simulink model "OtterFullForLqr_PositionControll_backup_LQR"  (R2020b)
settings: Solver=VariableStepAuto  StartTime=0.0  StopTime=30  RelTol=1e-3
values from neighbouring files (symbols this model uses):
  N = inv(Dcgain)    [LinMod60rpmForLqr.m]
  u0 = [60 60]'    [LinMod60rpmForLqr.m]
  x0 = OpTrim60.states.x    [LinMod60rpmForLqr.m]
undefined symbols (not defined in the file or in its folder): F
libraries: simulink x1, mssSimulink x1
settings Model: Creator=rapha  LastModifiedBy=rapha
settings DataIOCC: ExternalInput=getinputstruct(op_trim1)  InitialState=getstatestruct(op_trim1)

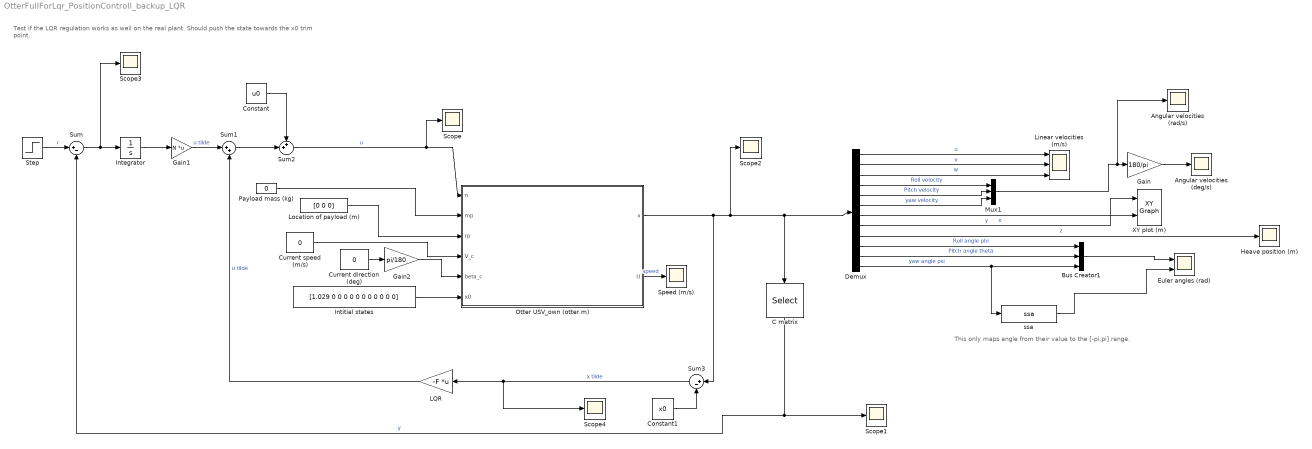
== system OtterFullForLqr_PositionControll_backup_LQR ==
  note: Test if the LQR regulation works as well on the real plant. Should push the state towards the x0 trim point.
  note: This only maps angle from their value to the [-pi,pi] range.
  Angular velocities (deg/s) : Scope
  Angular velocities (rad/s) : Scope
  Bus Creator1 : BusCreator  Inputs=3
  C matrix : Selector  InputPortWidth=12  IndexOptions=Index vector (dialog)  Indices=[1 6]  OutputSizes=1
  Constant : Constant  Value=u0
  Constant1 : Constant  Value=x0
  Current direction (deg) : Constant  Value=0
  Current speed (m/s) : Constant  Value=0
  Demux : Demux  Outputs=12
  Euler angles (rad) : Scope  NumInputPorts=2
  Gain : Gain  Gain=180/pi
  Gain1 : Gain  Gain=N  Multiplication=Matrix(K*u)
  Gain2 : Gain  Gain=pi/180
  Heave position (m) : Scope
  Integrator : Integrator
  Intitial states : Constant  Value=[1.029 0 0 0 0 0 0 0 0 0 0 0]
  LQR : Gain  Gain=-F  Multiplication=Matrix(K*u)
  Linear velocities (m/s) : Scope  NumInputPorts=3
  Location of payload (m) : Constant  Value=[0 0 0]
  Mux1 : Mux  Inputs=3
  "Otter USV_own (otter.m) " : Subsystem  AncestorBlock=mssSimulink/Marine craft models/Otter USV (otter.m)
      mask Display: image('otter.jpg'); % Use "Edit Image" on toolstrip to change.
  Payload mass (kg) : Constant  Value=0
  Scope{,1..4} (5 alike) : Scope
  Speed (m/s) : Scope
  Step : Step  Time=4  Before=[1.029 0]  After=[2 0.15]  SampleTime=0
  Sum : Sum  Inputs=|+-
  Sum1 : Sum  Inputs=|++
  Sum2 : Sum  Inputs=++|
  Sum3 : Sum  Inputs=|+-
  XY plot (m) : simulink/Sinks/XY Graph  xmin=-70  xmax=70  ymin=-70  ymax=70  st=0.01
  "ssa   " : mssSimulink/Utilities/Math Operations/ssa  SystemSampleTime=-1  VariantActivationTime=update diagram  Latency=0  AutoFrameSizeCalculation=off
  wires:
  Intitial states/1 -> "Otter USV_own (otter.m) "/6(x0)
  Payload mass (kg)/1 -> "Otter USV_own (otter.m) "/2(mp)
  Gain2/1 -> "Otter USV_own (otter.m) "/5(beta_c)
  Current direction (deg)/1 -> Gain2/1
  "Otter USV_own (otter.m) "/2(U) -> Speed (m/s)/1  "speed"
  Current speed (m/s)/1 -> "Otter USV_own (otter.m) "/4(V_c)
  Location of payload (m)/1 -> "Otter USV_own (otter.m) "/3(rp)
  Demux/1 -> Linear velocities (m/s)/1  "u"
  Demux/8 -> XY plot (m)/1  "y"
  Demux/7 -> XY plot (m)/2  "x"
  Demux/2 -> Linear velocities (m/s)/2  "v"
  Demux/3 -> Linear velocities (m/s)/3  "w"
  Gain/1 -> Angular velocities (deg/s)/1
  Mux1/1 -> Angular velocities (rad/s)/1, Gain/1
  Demux/4 -> Mux1/1  "Roll velocity"
  Demux/5 -> Mux1/2  "Pitch velocity"
  Demux/6 -> Mux1/3  "yaw velocity"
  Demux/9 -> Heave position (m)/1  "z"
  Demux/11 -> Bus Creator1/2  "Pitch angle theta"
  Bus Creator1/1 -> Euler angles (rad)/1
  Demux/10 -> Bus Creator1/1  "Roll angle phi"
  Demux/12 -> "ssa   "/1, Bus Creator1/3  "yaw angle psi"
  "ssa   "/1 -> Euler angles (rad)/2
  "Otter USV_own (otter.m) "/1(x) -> Sum3/1, C matrix/1, Demux/1, Scope2/1
  C matrix/1 -> Scope1/1, Sum/2  "y"
  Step/1 -> Sum/1  "r"
  Sum/1 -> Integrator/1, Scope3/1
  LQR/1 -> Sum1/2  "u tilde"
  Gain1/1 -> Sum1/1  "u tilde"
  Sum1/1 -> Sum2/2
  Sum2/1 -> Scope/1, "Otter USV_own (otter.m) "/1(n)  "u"
  Sum3/1 -> Scope4/1, LQR/1  "x tilde"
  Constant1/1 -> Sum3/2
  Constant/1 -> Sum2/1
  Integrator/1 -> Gain1/1

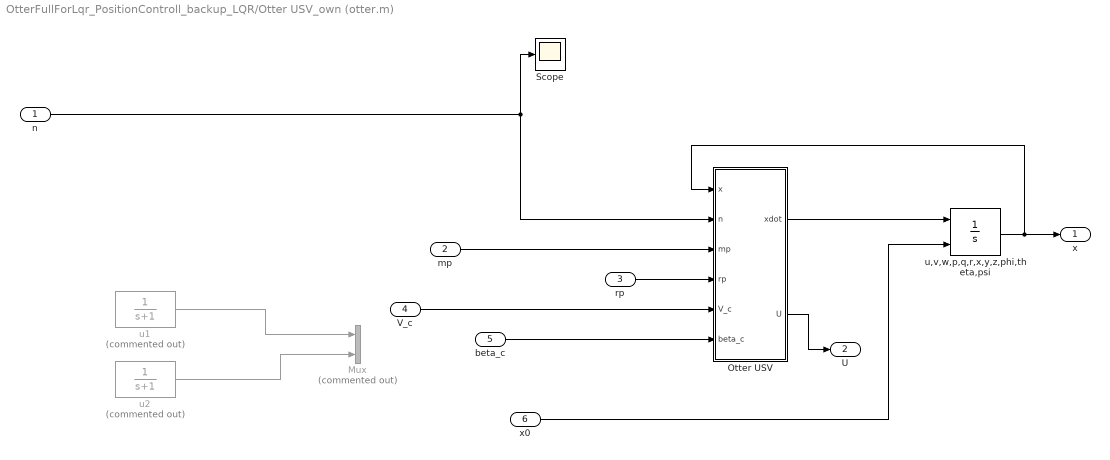
== system OtterFullForLqr_PositionControll_backup_LQR/Otter USV_own (otter.m)  ==
  n : Inport
  mp : Inport  Port=2
  rp : Inport  Port=3
  V_c : Inport  Port=4
  beta_c : Inport  Port=5
  x0 : Inport  Port=6
  Mux : Mux  Commented=on  Inputs=2
  Otter USV : MATLAB Function  TreatAsAtomicUnit=on
  Scope : Scope
  u,v,w,p,q,r,x,y,z,phi,theta,psi : Integrator  InitialConditionSource=external  InitialCondition=[1 1]  UpperSaturationLimit=10  LowerSaturationLimit=-10  AbsoluteTolerance=1e-3
  u1 : TransferFcn  Commented=on  Denominator=[1 1]
  u2 : TransferFcn  Commented=on  Denominator=[1 1]
  x : Outport
  U : Outport  Port=2
  wires:
  V_c/1 -> Otter USV/5(V_c)
  Otter USV/2(U) -> U/1
  mp/1 -> Otter USV/3(mp)
  Otter USV/1(xdot) -> u,v,w,p,q,r,x,y,z,phi,theta,psi/1
  u,v,w,p,q,r,x,y,z,phi,theta,psi/1 -> Otter USV/1(x), x/1
  beta_c/1 -> Otter USV/6(beta_c)
  rp/1 -> Otter USV/4(rp)
  x0/1 -> u,v,w,p,q,r,x,y,z,phi,theta,psi/2
  n/1 -> Scope/1, Otter USV/2(n)
  u2/1 -> Mux/2
  u1/1 -> Mux/1

== matlab function OtterFullForLqr_PositionControll_backup_LQR/Otter USV_own (otter.m) /Otter USV ==
  settings: updateMethod=DISCRETE
  data: x input; n input; xdot output; mp input; rp input; V_c input; beta_c input; U output
function [xdot,U] = fcn(x,n,mp,rp,V_c,beta_c)

[xdot,U] = OtterFunction_lqr(x,n,mp,rp,V_c,beta_c);

end
